simulink model "IntegratedControllerV9_WORKING"  (R2024b)
settings: Solver=FixedStepDiscrete  StartTime=0.0  StopTime=inf  FixedStep=0.01  RelTol=1e-3  EnableMultiTasking=on
model workspace (MAT data in the model file):
  kp = 1
undefined symbols (not defined in the file): a, b, dspDeleteFVToolLinkFromMask, gcbh
libraries: raspberrypiBasiclib x6, slpidlib x5, simulink x3, raspberrypiIOTlib x3, dspstat3 x2, etargetslib x2, eeGeneralControl x2, dspfiltersrcs x1
settings Model: ExtModeTrigDuration=2  Creator=alexs  LastModifiedBy=alexs
settings SolverCC: PositivePriorityOrder=on
settings OptimizationCC: EnhancedBackFolding=on  PassReuseOutputArgsAs=Individual arguments  ZeroExternalMemoryAtStartup=off  ZeroInternalMemoryAtStartup=off  MaxStackSize=200000  OptimizeBlockOrder=speed  DifferentSizesBufferReuse=on  EfficientTunableParamExpr=on
settings DebuggingCC: ParameterTunabilityLossMsg=error
settings HardwareCC: ProdBitPerPointer=32  ProdBitPerSizeT=32  ProdBitPerPtrDiffT=32  ProdLargestAtomicInteger=Long  ProdLargestAtomicFloat=Double  ProdWordSize=32  ProdLongLongMode=on  ProdHWDeviceType=ARM Compatible->ARM Cortex-A (32-bit)
settings RTWCC: Description=Embedded Coder  SystemTargetFile=ert.tlc  HardwareBoard=Raspberry Pi  TLCOptions="-aInlineSetEventsForThisBaseRateFcn=TLC_FALSE -aSuppressMultiTaskScheduler=TLC_FALSE  -aRateBasedStepFcn=0"  TemplateMakefile=ert_default_tmf  Toolchain=GNU GCC Embedded Linux  BuildConfiguration=Faster Runs
settings CodeAppCC: ForceParamTrailComments=on  IgnoreCustomStorageClasses=off  OperatorAnnotations=on  SimulinkDataObjDesc=on  SFDataObjDesc=on  InsertBlockDesc=on
settings ERTTargetCC: CodeReplacementLibrary=ARM Cortex-A CMSIS  SupportVariableSizeSignals=on  ExtModeTransport=2  ExtModeStaticAlloc=on  ExtModeMexFile=ext_xcp  ExtModeIntrfLevel=Level2 - Open  InlinedParameterPlacement=Hierarchical

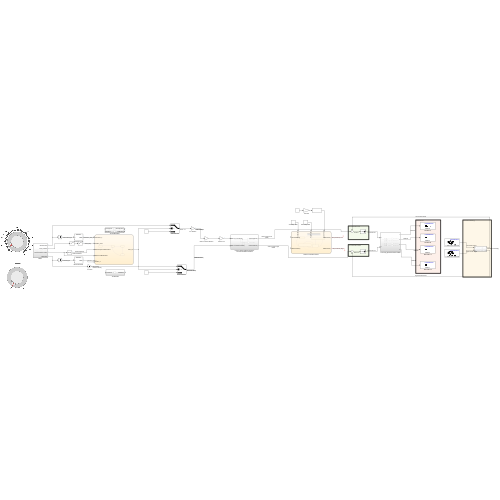
[thumbnail: Simulink's stored preview of the top-level diagram]
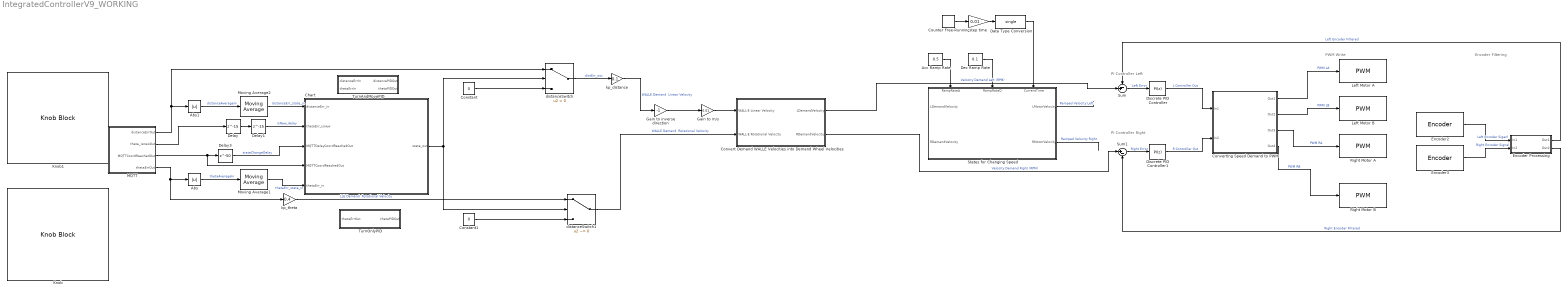
== system IntegratedControllerV9_WORKING ==
  note: PI Controller Right
  note: PWM Write
  note: PI Controller Left
  note: Encoder Filtering
  Abs : Abs  SaturateOnIntegerOverflow=off
  Abs1 : Abs  SaturateOnIntegerOverflow=off
  Acc Ramp Rate : Constant  Value=0.5  OutDataTypeStr=single
  Chart : Stateflow chart  TreatAsAtomicUnit=on
      settings: PortSchema="{\"entries\":[{\"content\":{\"sides\":[{\"content\":{\"connectorIds\":[\"In2\",\"In5\",\"In4\",\"In3\",\"In1\"]},\"type\":\"ConnectorPlacement.EquallySpacedRectSide\",\"uuid\":\"3dab0a91-9335-4990-9001-e160d82c945d\"},{\"content\":{\"connectorIds\":[\"Out1\"],\"side\":\"RIGHT\"},\"type\":\"ConnectorPlacement.EquallySpacedRectSide\",\"uuid\":\"b7b74537-0e0f-4d24-ad6a-0417436d6279\"},{\"content\":{\"side\":\"TOP\"},\"type\":\"ConnectorPlacement.EquallySpacedRectSide\",\"uuid\":\"7a696c29-7520-49e4-ace4-9e1abb82cb02\"}]},\"type\":\"ConnectorPlacement.EquallySpacedConnector\",\"uuid\":\"f02ffd70-1b39-4b11-b25b-86965795cc2a\"}],\"packageUris\":[\"http://schema.mathworks.com/mf0/Connector/R2020b\"],\"version\":\"1.0\"}"
  Constant : Constant  Value=0
  Constant1 : Constant  Value=0
  Convert Demand WALLE Velocities into Demand Wheel Velocities : Subsystem
  Converting Speed Demand to PWM : Subsystem
  Counter Free-Running : simulink/Sources/Counter Free-Running  NumBits=16  tsamp=-1
  Data Type Conversion : DataTypeConversion  OutDataTypeStr=single  SaturateOnIntegerOverflow=off  RndMeth=Floor
  Dec Ramp Rate : Constant  Value=0.1  OutDataTypeStr=single
  Delay : Delay  DelayLength=15  InitialCondition=0
  Delay1 : Delay  DelayLength=15  InitialCondition=0
  Delay3 : Delay  DelayLength=50  InitialCondition=0
  Discrete PID Controller : slpidlib/PID Controller  Controller=PI  Form=Parallel  TimeDomain=Discrete-time  UseExternalTs=off  SampleTime=-1  IntegratorMethod=Forward Euler  FilterMethod=Forward Euler  ControllerParametersSource=internal  P=1.7  I=0.4  UseKiTs=off  D=0.001  UseExternalDerivativeSource=off  N=100  UseFilter=on  TunerSelectOption=Transfer Function Based (PID Tuner App)  InitialConditionSource=internal  InitialConditionForIntegrator=0  InitialConditionForFilter=0  DifferentiatorICPrevScaledInput=0  ExternalReset=none  TrackingMode=off  Kt=1  LimitOutput=on  SatLimitsSource=internal  UpperSaturationLimit=44  LowerSaturationLimit=-44  LinearizeAsGain=off  AntiWindupMode=none  Kb=1  LimitIntegrator=off  UpperIntegratorSaturationLimit=inf  LowerIntegratorSaturationLimit=-inf  POutMin=[]  POutMax=[]  IOutMin=[]  IOutMax=[]  DOutMin=[]  DOutMax=[]  NOutMin=[]  NOutMax=[]  SumOutDataTypeStr=single  SumOutMin=[]  SumOutMax=[]  SaturationOutMin=[]  SaturationOutMax=[]  PParamMin=[]  PParamMax=[]  IParamMin=[]  IParamMax=[]  DParamMin=[]  DParamMax=[]  NParamMin=[]  NParamMax=[]  KbParamMin=[]  KbParamMax=[]  KtParamMin=[]  KtParamMax=[]  KbOutMin=[]  KbOutMax=[]  KtOutMin=[]  KtOutMax=[]  IntegratorOutMin=[]  IntegratorOutMax=[]  FilterOutMin=[]  FilterOutMax=[]  SumI1OutMin=[]  SumI1OutMax=[]  SumI2OutMin=[]  SumI2OutMax=[]  SumI3OutMin=[]  SumI3OutMax=[]  SumI4OutMin=[]  SumI4OutMax=[]  SumDOutMin=[]  SumDOutMax=[]  DifferentiatorOutMin=[]  DifferentiatorOutMax=[]  FilterDiffOutCoefMin=[]  FilterDiffOutCoefMax=[]  ReciprocalOutMin=[]  ReciprocalOutMax=[]  SumDenOutMin=[]  SumDenOutMax=[]  SumNumOutMin=[]  SumNumOutMax=[]  DivideOutMin=[]  DivideOutMax=[]  UdiffTsProdOutMin=[]  UdiffTsProdOutMax=[]  NTsProdOutMin=[]  NTsProdOutMax=[]  UintegralTsProdOutMin=[]  UintegralTsProdOutMax=[]  UngainTsProdOutMin=[]  UngainTsProdOutMax=[]  ClampingZeroOutDataTypeStr=Inherit: Inherit via back propagation  ClampingZeroOutMin=[]  ClampingZeroOutMax=[]  FilterDenConstantOutDataTypeStr=Inherit: Inherit via back propagation  FilterDenConstantOutMin=[]  FilterDenConstantOutMax=[]  PCopyOutDataTypeStr=Inherit: Inherit via back propagation  PCopyOutMin=[]  PCopyOutMax=[]  NCopyOutDataTypeStr=Inherit: Inherit via back propagation  NCopyOutMin=[]  NCopyOutMax=[]  IntegratorContinuousStateAttributes=''  IntegratorStateMustResolveToSignalObject=off  IntegratorRTWStateStorageClass=Auto  FilterContinuousStateAttributes=''  FilterStateMustResolveToSignalObject=off  FilterRTWStateStorageClass=Auto  ParallelPVariant=InternalParameters  IdealPVariant=Disabled  IVariant=InternalParameters  DVariant=Disabled  IntegratorVariant=Discrete  SatVariant=Enabled  AWVariant=Passthrough  PCopyVariant=Disabled  TRVariant=Disabled  FdbkBlocksVariant=Forward  IdealPFdbkVariant=Disabled  SatFdbkVariant=Disabled  DerivativeFilterVariant=Disabled  NVariant=Disabled  NCopyVariant=Disabled_SignalSpec  FilterICVariant=Disabled  IntegratorICVariant=InternalICs  ExternalResetVariant=Disabled  TRSumVariant=Passthrough  SumFdbkVariant=Disabled  SumVariant=Sum_PI  TsampFilterVariant=InternalTs  TsampNgainVariant=Passthrough  TsampIntegralVariant=Disabled_SignalSpec  ExternalSaturationOutDataTypeStr=Inherit: Same as second input  DerivativeSourceVariant=Disabled  PreIntVariant=InternalPreInt
      settings: LibrarySourceBlock=simulink/Discrete/Discrete PID Controller
  Discrete PID Controller1 : slpidlib/PID Controller  Controller=PI  Form=Parallel  TimeDomain=Discrete-time  UseExternalTs=off  SampleTime=-1  IntegratorMethod=Forward Euler  FilterMethod=Forward Euler  ControllerParametersSource=internal  P=1.7  I=0.4  UseKiTs=off  D=0  UseExternalDerivativeSource=off  N=100  UseFilter=on  TunerSelectOption=Transfer Function Based (PID Tuner App)  InitialConditionSource=internal  InitialConditionForIntegrator=0  InitialConditionForFilter=0  DifferentiatorICPrevScaledInput=0  ExternalReset=none  TrackingMode=off  Kt=1  LimitOutput=on  SatLimitsSource=internal  UpperSaturationLimit=44  LowerSaturationLimit=-44  LinearizeAsGain=off  AntiWindupMode=none  Kb=1  LimitIntegrator=off  UpperIntegratorSaturationLimit=inf  LowerIntegratorSaturationLimit=-inf  POutMin=[]  POutMax=[]  IOutMin=[]  IOutMax=[]  DOutMin=[]  DOutMax=[]  NOutMin=[]  NOutMax=[]  SumOutMin=[]  SumOutMax=[]  SaturationOutMin=[]  SaturationOutMax=[]  PParamMin=[]  PParamMax=[]  IParamMin=[]  IParamMax=[]  DParamMin=[]  DParamMax=[]  NParamMin=[]  NParamMax=[]  KbParamMin=[]  KbParamMax=[]  KtParamMin=[]  KtParamMax=[]  KbOutMin=[]  KbOutMax=[]  KtOutMin=[]  KtOutMax=[]  IntegratorOutMin=[]  IntegratorOutMax=[]  FilterOutMin=[]  FilterOutMax=[]  SumI1OutMin=[]  SumI1OutMax=[]  SumI2OutMin=[]  SumI2OutMax=[]  SumI3OutMin=[]  SumI3OutMax=[]  SumI4OutMin=[]  SumI4OutMax=[]  SumDOutMin=[]  SumDOutMax=[]  DifferentiatorOutMin=[]  DifferentiatorOutMax=[]  FilterDiffOutCoefMin=[]  FilterDiffOutCoefMax=[]  ReciprocalOutMin=[]  ReciprocalOutMax=[]  SumDenOutMin=[]  SumDenOutMax=[]  SumNumOutMin=[]  SumNumOutMax=[]  DivideOutMin=[]  DivideOutMax=[]  UdiffTsProdOutMin=[]  UdiffTsProdOutMax=[]  NTsProdOutMin=[]  NTsProdOutMax=[]  UintegralTsProdOutMin=[]  UintegralTsProdOutMax=[]  UngainTsProdOutMin=[]  UngainTsProdOutMax=[]  ClampingZeroOutDataTypeStr=Inherit: Inherit via back propagation  ClampingZeroOutMin=[]  ClampingZeroOutMax=[]  FilterDenConstantOutDataTypeStr=Inherit: Inherit via back propagation  FilterDenConstantOutMin=[]  FilterDenConstantOutMax=[]  PCopyOutDataTypeStr=Inherit: Inherit via back propagation  PCopyOutMin=[]  PCopyOutMax=[]  NCopyOutDataTypeStr=Inherit: Inherit via back propagation  NCopyOutMin=[]  NCopyOutMax=[]  IntegratorContinuousStateAttributes=''  IntegratorStateMustResolveToSignalObject=off  IntegratorRTWStateStorageClass=Auto  FilterContinuousStateAttributes=''  FilterStateMustResolveToSignalObject=off  FilterRTWStateStorageClass=Auto  ParallelPVariant=InternalParameters  IdealPVariant=Disabled  IVariant=InternalParameters  DVariant=Disabled  IntegratorVariant=Discrete  SatVariant=Enabled  AWVariant=Passthrough  PCopyVariant=Disabled  TRVariant=Disabled  FdbkBlocksVariant=Forward  IdealPFdbkVariant=Disabled  SatFdbkVariant=Disabled  DerivativeFilterVariant=Disabled  NVariant=Disabled  NCopyVariant=Disabled_SignalSpec  FilterICVariant=Disabled  IntegratorICVariant=InternalICs  ExternalResetVariant=Disabled  TRSumVariant=Passthrough  SumFdbkVariant=Disabled  SumVariant=Sum_PI  TsampFilterVariant=InternalTs  TsampNgainVariant=Passthrough  TsampIntegralVariant=Disabled_SignalSpec  ExternalSaturationOutDataTypeStr=Inherit: Same as second input  DerivativeSourceVariant=Disabled  PreIntVariant=InternalPreInt
      settings: LibrarySourceBlock=simulink/Discrete/Discrete PID Controller
  Encoder Processing : Subsystem
  Encoder2 : raspberrypiBasiclib/Encoder  BoardProperty=Pi 3 Model B+  InputA=GPIO 16  InputB=GPIO 20  Mode=No reset  SampleTime=-1
  Encoder3 : raspberrypiBasiclib/Encoder  BoardProperty=Pi 3 Model B+  InputA=GPIO 19  InputB=GPIO 26  Mode=No reset  SampleTime=-1
  Gain to inverse direction : Gain  Gain=-1
  Gain to m/s : Gain  Gain=0.01
  Knob : KnobBlock  ScaleMin=0.4  ScaleMax=0.8  ScaleType=Log
  Knob1 : KnobBlock  ScaleMax=1
  Left Motor A : raspberrypiBasiclib/PWM  board=Pi 3 Model B+  Pin_=18  Frequency=4000  blockPlatform=Raspberry Pi
  Left Motor B : raspberrypiBasiclib/PWM  board=Pi 3 Model B+  Pin_=14  Frequency=4000  blockPlatform=Raspberry Pi
  MQTT : Subsystem
  Moving Average1 : eeGeneralControl/Moving Average  VariantControl=Variant1  LabelModeActiveChoice=Discrete  f=1  x0=10  BufferSize=8192  Ts=-1
      settings: LibrarySourceBlock=ee_sl_lib/General Control/Moving Average
  Moving Average2 : eeGeneralControl/Moving Average  VariantControl=Variant1  LabelModeActiveChoice=Discrete  f=1  x0=10  BufferSize=8192  Ts=-1
      settings: LibrarySourceBlock=ee_sl_lib/General Control/Moving Average
  Right Motor A : raspberrypiBasiclib/PWM  board=Pi 3 Model B+  Pin_=27  Frequency=4000  blockPlatform=Raspberry Pi
  Right Motor B : raspberrypiBasiclib/PWM  board=Pi 3 Model B+  Pin_=17  Frequency=4000  blockPlatform=Raspberry Pi
  States for Changing Speed : Stateflow chart  TreatAsAtomicUnit=on
      settings: PortSchema="{\"entries\":[{\"content\":{\"sides\":[{\"content\":{\"connectorIds\":[\"In1\",\"In2\"]},\"type\":\"ConnectorPlacement.EquallySpacedRectSide\",\"uuid\":\"29566149-d476-48be-bb8d-fc9ab2ff4a55\"},{\"content\":{\"connectorIds\":[\"Out1\",\"Out2\"],\"side\":\"RIGHT\"},\"type\":\"ConnectorPlacement.EquallySpacedRectSide\",\"uuid\":\"f908ad7a-2ba5-4204-8f83-b7448630d8f9\"},{\"content\":{\"connectorIds\":[\"In3\",\"In4\",\"In5\"],\"side\":\"TOP\"},\"type\":\"ConnectorPlacement.EquallySpacedRectSide\",\"uuid\":\"1bf600d9-c304-4bcd-9fe1-9d209939bb1c\"}]},\"type\":\"ConnectorPlacement.EquallySpacedConnector\",\"uuid\":\"d153a689-9e68-4d3b-a6cb-2781800d561b\"}],\"packageUris\":[\"http://schema.mathworks.com/mf0/Connector/R2020b\"],\"version\":\"1.0\"}"
  Sum : Sum  Inputs=-+|
  Sum1 : Sum  Inputs=|+-
  TurnAndMovePID : Subsystem
  TurnOnlyPID : Subsystem
  distanceSwitch : Switch  Criteria=u2 > Threshold  SaturateOnIntegerOverflow=off  InputSameDT=off
  distanceSwitch1 : Switch  Criteria=u2 ~= 0  SaturateOnIntegerOverflow=off  InputSameDT=off
  kp_distance : Gain  Gain=0.1
  kp_theta : Gain  Gain=0.4
  step time : Gain  Gain=0.01
  wires:
  distanceSwitch1/1 -> Convert Demand WALLE Velocities into Demand Wheel Velocities/2(WALL-E Rotational Velocity)  "WALLE Demand  Rotational Velocity"
  Discrete PID Controller/1 -> Converting Speed Demand to PWM/1(In1)  "L Controller Out"
  Converting Speed Demand to PWM/1(Out1) -> Left Motor A/1  "PWM LA"
  Encoder3/1 -> Encoder Processing/2(In2)  "Right Encoder Signal"
  Counter Free-Running/1 -> step time/1
  Sum1/1 -> Discrete PID Controller1/1  "Right Error"
  step time/1 -> Data Type Conversion/1
  States for Changing Speed/2(RMotorVelocity) -> ?  "Ramped Velocity Right"
  Converting Speed Demand to PWM/3(Out3) -> Right Motor A/1  "PWM RA"
  Encoder2/1 -> Encoder Processing/1(In1)  "Left Encoder Siganl"
  Encoder Processing/2(Out2) -> Sum1/2  "Right Encoder Filtered"
  Discrete PID Controller1/1 -> Converting Speed Demand to PWM/2(In2)  "R Controller Out"
  kp_distance/1 -> Gain to inverse direction/1  "WALLE Demand  Linear Velocity"
  Sum/1 -> Discrete PID Controller/1  "Left Error"
  Converting Speed Demand to PWM/4(Out4) -> Right Motor B/1  "PWM RB"
  Acc Ramp Rate/1 -> States for Changing Speed/3(RampRateA)
  Data Type Conversion/1 -> States for Changing Speed/5(CurrentTime)
  States for Changing Speed/1(LMotorVelocity) -> ?  "Ramped Velocity Left"
  Convert Demand WALLE Velocities into Demand Wheel Velocities/1(LDemandVelocity) -> Sum/2  "Velocity Demand Left (RPM)"
  Encoder Processing/1(Out1) -> Sum/1  "Left Encoder Filtered"
  Converting Speed Demand to PWM/2(Out2) -> Left Motor B/1  "PWM LB"
  Dec Ramp Rate/1 -> States for Changing Speed/4(RampRateD)
  Convert Demand WALLE Velocities into Demand Wheel Velocities/2(RDemandVelocity) -> Sum1/1  "Velocity Demand Right (RPM)"
  MQTT/1(distanceErrOut) -> distanceSwitch/1, Abs1/1
  Constant/1 -> distanceSwitch/3
  MQTT/4(thetaErrOut) -> Abs/1, kp_theta/1
  Chart/1(state_out) -> distanceSwitch1/2, distanceSwitch/2
  Abs1/1 -> Moving Average2/1  "distanceAverageIn"
  Abs/1 -> Moving Average1/1  "thetaAverageIn"
  distanceSwitch/1 -> kp_distance/1  "distErr_out"
  Moving Average1/1 -> Chart/1(thetaErr_in)  "thetaErr_state_in"
  Moving Average2/1 -> Chart/2(distanceErr_in)  "distanceErr_state_in"
  Delay/1 -> Delay1/1
  MQTT/2(theta_isnewOut) -> Delay/1
  Delay1/1 -> Chart/5(thetaErr_isnew)  "isNew_delay"
  Gain to inverse direction/1 -> Gain to m/s/1
  Gain to m/s/1 -> Convert Demand WALLE Velocities into Demand Wheel Velocities/1(WALL-E Linear Velocity)
  kp_theta/1 -> distanceSwitch1/1  "LLE Demand  Rotational Velocity"
  Constant1/1 -> distanceSwitch1/3
  MQTT/3(MQTTCoordReachedOut) -> Chart/3(MQTTCoordReachedOut), Delay3/1
  Delay3/1 -> Chart/4(MQTTDelayCoordReachedOut)  "stateChangeDelay"

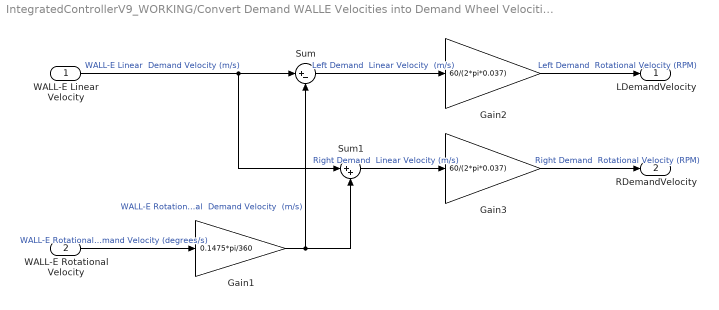
== system IntegratedControllerV9_WORKING/Convert Demand WALLE Velocities into Demand Wheel Velocities ==
  WALL-E Linear Velocity : Inport
  WALL-E Rotational Velocity : Inport  Port=2
  Gain1 : Gain  Gain=0.1475*pi/360
  Gain2 : Gain  Gain=60/(2*pi*0.037)
  Gain3 : Gain  Gain=60/(2*pi*0.037)
  Sum : Sum  Inputs=|+-  OutDataTypeStr=single
  Sum1 : Sum  Inputs=|++  OutDataTypeStr=single
  LDemandVelocity : Outport
  RDemandVelocity : Outport  Port=2
  wires:
  WALL-E Linear Velocity/1 -> Sum1/1, Sum/1  "WALL-E Linear  Demand Velocity (m/s)"
  WALL-E Rotational Velocity/1 -> Gain1/1  "WALL-E Rotational  Demand Velocity (degrees/s)"
  Gain1/1 -> Sum1/2, Sum/2  "WALL-E Rotational  Demand Velocity  (m/s)"
  Sum/1 -> Gain2/1  "Left Demand  Linear Velocity  (m/s)"
  Gain2/1 -> LDemandVelocity/1  "Left Demand  Rotational Velocity (RPM)"
  Sum1/1 -> Gain3/1  "Right Demand  Linear Velocity (m/s)"
  Gain3/1 -> RDemandVelocity/1  "Right Demand  Rotational Velocity (RPM)"

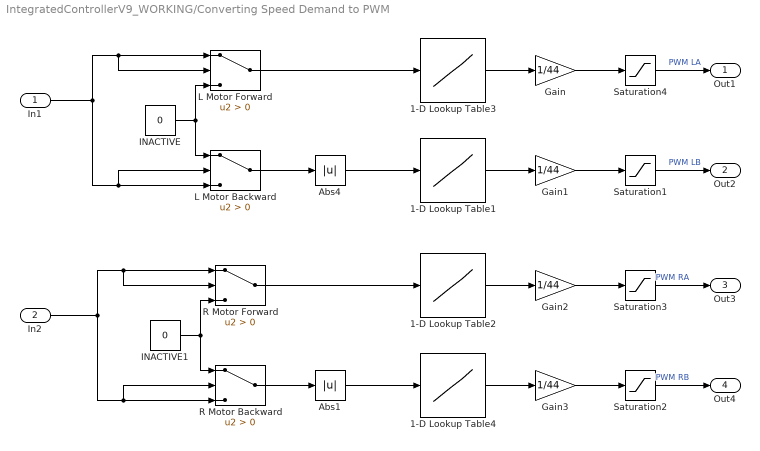
== system IntegratedControllerV9_WORKING/Converting Speed Demand to PWM ==
  In1 : Inport
  In2 : Inport  Port=2
  1-D Lookup Table{1..4} (4 alike) : Lookup_n-D  NumberOfTableDimensions=1  BreakpointsForDimension1=[0 2.1000000000000001 3.7000000000000002 5 10 15 20 25 30 35 40]  Table=[0 0 3.7000000000000002 3.7999999999999998 5 6 7 8 9 12 25]  InternalRulePriority=Speed  RndMeth=Simplest
  Abs1 : Abs  SaturateOnIntegerOverflow=off
  Abs4 : Abs  SaturateOnIntegerOverflow=off
  Gain{,1..3} (4 alike) : Gain  Gain=1/44
  INACTIVE : Constant  Value=0
  INACTIVE1 : Constant  Value=0
  L Motor Backward : Switch  Criteria=u2 > Threshold  SaturateOnIntegerOverflow=off  InputSameDT=off
  L Motor Forward : Switch  Criteria=u2 > Threshold  SaturateOnIntegerOverflow=off  InputSameDT=off
  R Motor Backward : Switch  Criteria=u2 > Threshold  SaturateOnIntegerOverflow=off  InputSameDT=off
  R Motor Forward : Switch  Criteria=u2 > Threshold  SaturateOnIntegerOverflow=off  InputSameDT=off
  Saturation{1..4} (4 alike) : Saturate  UpperLimit=1  LowerLimit=0
  Out1 : Outport
  Out2 : Outport  Port=2
  Out3 : Outport  Port=3
  Out4 : Outport  Port=4
  wires:
  L Motor Forward/1 -> 1-D Lookup Table3/1
  In1/1 -> L Motor Backward/2, L Motor Backward/3, L Motor Forward/2, L Motor Forward/1
  INACTIVE/1 -> L Motor Forward/3, L Motor Backward/1
  INACTIVE1/1 -> R Motor Forward/3, R Motor Backward/1
  R Motor Backward/1 -> Abs1/1
  In2/1 -> R Motor Backward/2, R Motor Backward/3, R Motor Forward/2, R Motor Forward/1
  R Motor Forward/1 -> 1-D Lookup Table2/1
  Saturation1/1 -> Out2/1  "PWM LB"
  Abs4/1 -> 1-D Lookup Table1/1
  L Motor Backward/1 -> Abs4/1
  Saturation4/1 -> Out1/1  "PWM LA"
  Saturation3/1 -> Out3/1  "PWM RA"
  Abs1/1 -> 1-D Lookup Table4/1
  Saturation2/1 -> Out4/1  "PWM RB"
  1-D Lookup Table2/1 -> Gain2/1
  1-D Lookup Table1/1 -> Gain1/1
  1-D Lookup Table3/1 -> Gain/1
  1-D Lookup Table4/1 -> Gain3/1
  Gain/1 -> Saturation4/1
  Gain1/1 -> Saturation1/1
  Gain2/1 -> Saturation3/1
  Gain3/1 -> Saturation2/1

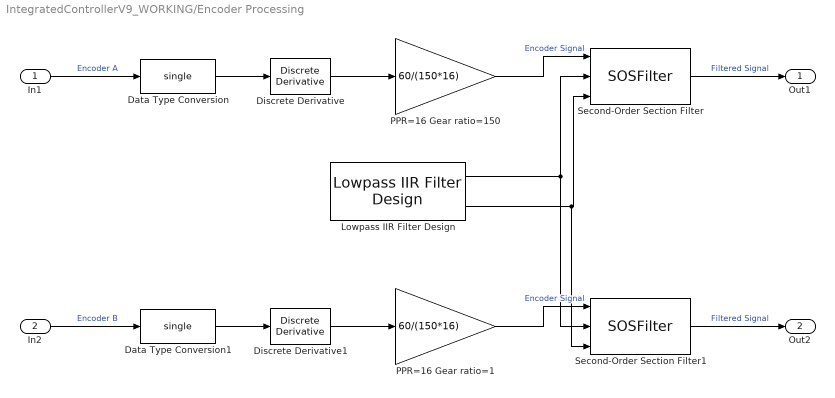
== system IntegratedControllerV9_WORKING/Encoder Processing ==
  In1 : Inport
  In2 : Inport  Port=2
  Data Type Conversion : DataTypeConversion  OutDataTypeStr=single  SaturateOnIntegerOverflow=off  RndMeth=Floor
  Data Type Conversion1 : DataTypeConversion  OutDataTypeStr=single  SaturateOnIntegerOverflow=off  RndMeth=Floor
  Discrete Derivative : simulink/Discrete/Discrete Derivative  gainval=1  ICPrevScaledInput=0.0  OutMin=[]  OutMax=[]  OutDataType=fixdt(1, 16)  OutScaling=2^-10  DoSatur=off
  Discrete Derivative1 : simulink/Discrete/Discrete Derivative  gainval=1  ICPrevScaledInput=0.0  OutMin=[]  OutMax=[]  OutDataType=fixdt(1, 16)  OutScaling=2^-10  DoSatur=off
  Lowpass IIR Filter Design : dspfiltersrcs/Lowpass IIR Filter Design  SmoothParameters=off  SmoothingFactor=0.6  DesignMethod=Butterworth  FilterOrderPort=off  FilterOrder=2  MaxOrder=2  F3dBPort=off  F3dB=50/200  ApassPort=off  Apass=1  AstopPort=off  Astop=60  HasScaleValues=off  OutputDataType=single  SampleTime=-1  SimulateUsing=Interpreted execution
  PPR=16 Gear ratio=1 : Gain  Gain=60/(150*16)  OutDataTypeStr=single
  PPR=16 Gear ratio=150 : Gain  Gain=60/(150*16)  OutDataTypeStr=single
  Second-Order Section Filter : SOSFilter  LoadFcn=dspDeleteFVToolLinkFromMask(gcbh);  CoeffSource=Input ports  Numerator=b  Denominator=a
      settings: DeleteFcn=dspLinkFVTool2Mask(gcbh,'close')  ModelCloseFcn=dspLinkFVTool2Mask(gcbh,'close')  PreSaveFcn=dspUnlinkFVToolFromMask(gcbh);  PostSaveFcn=dspRestoreLinkFVTool2Mask(gcbh);  CloseFcn=dspLinkFVTool2Mask(gcbh,'close')  InputPortMap=u0,u1,u2
      settings: CopyFcn=|
      | ud = get_param(gcbh,'UserData');
      | if isfield(ud,'fvtool')
      |   ud = rmfield(ud,'fvtool');
      |   set_param(gcbh,'UserData',ud);
      | end
      | clear ud
  Second-Order Section Filter1 : SOSFilter  LoadFcn=dspDeleteFVToolLinkFromMask(gcbh);  CoeffSource=Input ports  Numerator=b  Denominator=a
      settings: DeleteFcn=dspLinkFVTool2Mask(gcbh,'close')  ModelCloseFcn=dspLinkFVTool2Mask(gcbh,'close')  PreSaveFcn=dspUnlinkFVToolFromMask(gcbh);  PostSaveFcn=dspRestoreLinkFVTool2Mask(gcbh);  CloseFcn=dspLinkFVTool2Mask(gcbh,'close')  InputPortMap=u0,u1,u2
      settings: CopyFcn=|
      | ud = get_param(gcbh,'UserData');
      | if isfield(ud,'fvtool')
      |   ud = rmfield(ud,'fvtool');
      |   set_param(gcbh,'UserData',ud);
      | end
      | clear ud
  Out1 : Outport
  Out2 : Outport  Port=2
  wires:
  In1/1 -> Data Type Conversion/1  "Encoder A"
  Second-Order Section Filter/1 -> Out1/1  "Filtered Signal"
  Discrete Derivative/1 -> PPR=16 Gear ratio=150/1
  PPR=16 Gear ratio=150/1 -> Second-Order Section Filter/1  "Encoder Signal"
  Data Type Conversion/1 -> Discrete Derivative/1
  Lowpass IIR Filter Design/2 -> Second-Order Section Filter1/3, Second-Order Section Filter/3
  Data Type Conversion1/1 -> Discrete Derivative1/1
  PPR=16 Gear ratio=1/1 -> Second-Order Section Filter1/1  "Encoder Signal"
  Second-Order Section Filter1/1 -> Out2/1  "Filtered Signal"
  Discrete Derivative1/1 -> PPR=16 Gear ratio=1/1
  In2/1 -> Data Type Conversion1/1  "Encoder B"
  Lowpass IIR Filter Design/1 -> Second-Order Section Filter/2, Second-Order Section Filter1/2

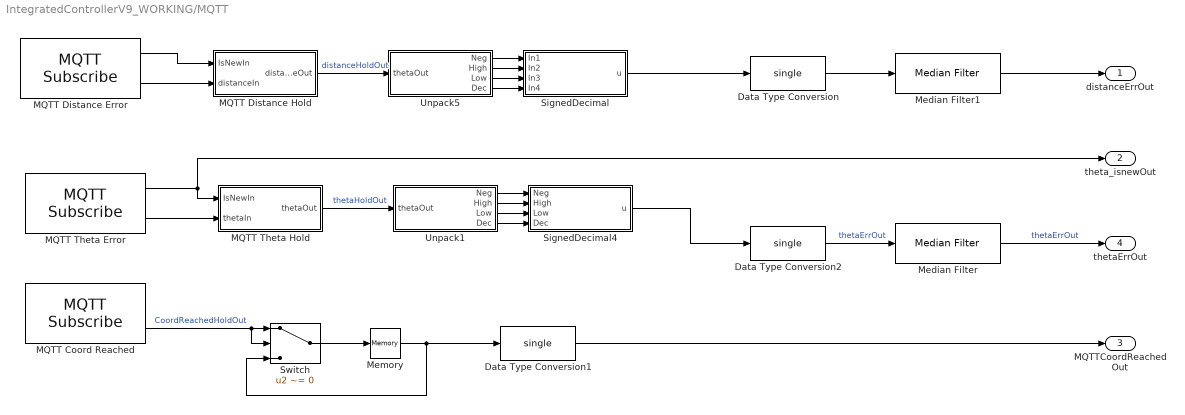
== system IntegratedControllerV9_WORKING/MQTT ==
  Data Type Conversion : DataTypeConversion  OutDataTypeStr=single  SaturateOnIntegerOverflow=off  RndMeth=Floor
  Data Type Conversion1 : DataTypeConversion  OutDataTypeStr=single  SaturateOnIntegerOverflow=off  RndMeth=Floor
  Data Type Conversion2 : DataTypeConversion  OutDataTypeStr=single  SaturateOnIntegerOverflow=off  RndMeth=Floor
  MQTT Coord Reached : raspberrypiIOTlib/MQTT Subscribe  Topic=Wall-E/position_controller/coord_reached  QoS=2  MessageLength=1  OutputMessage=on  SampleTime=.05  blockPlatform=RASPBERRYPI
  MQTT Distance Error : raspberrypiIOTlib/MQTT Subscribe  Topic=Wall-E/position_controller/error/dist  QoS=2  MessageLength=4  OutputMessage=on  SampleTime=.05  blockPlatform=RASPBERRYPI
  MQTT Distance Hold : Subsystem
  MQTT Theta Error : raspberrypiIOTlib/MQTT Subscribe  Topic=Wall-E/position_controller/error/theta  QoS=2  MessageLength=4  OutputMessage=on  SampleTime=.05  blockPlatform=RASPBERRYPI
  MQTT Theta Hold : Subsystem
  Median Filter : dspstat3/Median Filter  WindowLength=8  SimulateUsing=Interpreted execution
      settings: LibrarySourceBlock=|
      | dspfdesign/Median
      | Filter
  Median Filter1 : dspstat3/Median Filter  WindowLength=8  SimulateUsing=Interpreted execution
      settings: LibrarySourceBlock=|
      | dspfdesign/Median
      | Filter
  Memory : Memory  InheritSampleTime=on
  SignedDecimal : Subsystem
  SignedDecimal4 : Subsystem
  Switch : Switch  Criteria=u2 ~= 0  SaturateOnIntegerOverflow=off  InputSameDT=off
  Unpack1 : Subsystem
  Unpack5 : Subsystem
  distanceErrOut : Outport
  theta_isnewOut : Outport  Port=2
  MQTTCoordReachedOut : Outport  Port=3
  thetaErrOut : Outport  Port=4
  wires:
  Unpack5/4(Dec) -> SignedDecimal/4(In4)
  Unpack5/1(Neg) -> SignedDecimal/1(In1)
  Unpack5/2(High) -> SignedDecimal/2(In2)
  SignedDecimal/1(u) -> Data Type Conversion/1
  Unpack5/3(Low) -> SignedDecimal/3(In3)
  Median Filter1/1 -> distanceErrOut/1
  Unpack1/1(Neg) -> SignedDecimal4/1(Neg)
  Unpack1/2(High) -> SignedDecimal4/2(High)
  Unpack1/3(Low) -> SignedDecimal4/3(Low)
  Unpack1/4(Dec) -> SignedDecimal4/4(Dec)
  SignedDecimal4/1(u) -> Data Type Conversion2/1
  Median Filter/1 -> thetaErrOut/1  "thetaErrOut"
  MQTT Theta Error/1 -> theta_isnewOut/1, MQTT Theta Hold/1(IsNewIn)
  MQTT Theta Hold/1(thetaOut) -> Unpack1/1(thetaOut)  "thetaHoldOut"
  MQTT Theta Error/2 -> MQTT Theta Hold/2(thetaIn)
  MQTT Distance Hold/1(distanceOut) -> Unpack5/1(thetaOut)  "distanceHoldOut"
  MQTT Distance Error/2 -> MQTT Distance Hold/2(distanceIn)
  MQTT Distance Error/1 -> MQTT Distance Hold/1(IsNewIn)
  Data Type Conversion2/1 -> Median Filter/1  "thetaErrOut"
  Data Type Conversion/1 -> Median Filter1/1
  Switch/1 -> Memory/1
  Memory/1 -> Data Type Conversion1/1, Switch/3
  MQTT Coord Reached/2 -> Switch/2, Switch/1  "CoordReachedHoldOut"
  Data Type Conversion1/1 -> MQTTCoordReachedOut/1

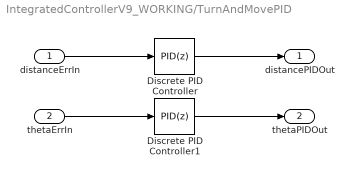
== system IntegratedControllerV9_WORKING/TurnAndMovePID ==
  distanceErrIn : Inport
  thetaErrIn : Inport  Port=2
  Discrete PID Controller : slpidlib/PID Controller  Controller=PID  Form=Parallel  TimeDomain=Discrete-time  UseExternalTs=off  SampleTime=0.25  IntegratorMethod=Forward Euler  FilterMethod=Forward Euler  ControllerParametersSource=internal  P=0.01  I=0  UseKiTs=off  D=.001  UseExternalDerivativeSource=off  N=100  UseFilter=on  TunerSelectOption=Transfer Function Based (PID Tuner App)  InitialConditionSource=internal  InitialConditionForIntegrator=0  InitialConditionForFilter=0  DifferentiatorICPrevScaledInput=0  ExternalReset=none  TrackingMode=off  Kt=1  LimitOutput=on  SatLimitsSource=internal  UpperSaturationLimit=1  LowerSaturationLimit=-1  LinearizeAsGain=off  AntiWindupMode=none  Kb=1  LimitIntegrator=off  UpperIntegratorSaturationLimit=inf  LowerIntegratorSaturationLimit=-inf  POutMin=[]  POutMax=[]  IOutMin=[]  IOutMax=[]  DOutMin=[]  DOutMax=[]  NOutMin=[]  NOutMax=[]  SumOutMin=[]  SumOutMax=[]  SaturationOutMin=[]  SaturationOutMax=[]  PParamMin=[]  PParamMax=[]  IParamMin=[]  IParamMax=[]  DParamMin=[]  DParamMax=[]  NParamMin=[]  NParamMax=[]  KbParamMin=[]  KbParamMax=[]  KtParamMin=[]  KtParamMax=[]  KbOutMin=[]  KbOutMax=[]  KtOutMin=[]  KtOutMax=[]  IntegratorOutMin=[]  IntegratorOutMax=[]  FilterOutMin=[]  FilterOutMax=[]  SumI1OutMin=[]  SumI1OutMax=[]  SumI2OutMin=[]  SumI2OutMax=[]  SumI3OutMin=[]  SumI3OutMax=[]  SumI4OutMin=[]  SumI4OutMax=[]  SumDOutMin=[]  SumDOutMax=[]  DifferentiatorOutMin=[]  DifferentiatorOutMax=[]  FilterDiffOutCoefMin=[]  FilterDiffOutCoefMax=[]  ReciprocalOutMin=[]  ReciprocalOutMax=[]  SumDenOutMin=[]  SumDenOutMax=[]  SumNumOutMin=[]  SumNumOutMax=[]  DivideOutMin=[]  DivideOutMax=[]  UdiffTsProdOutMin=[]  UdiffTsProdOutMax=[]  NTsProdOutMin=[]  NTsProdOutMax=[]  UintegralTsProdOutMin=[]  UintegralTsProdOutMax=[]  UngainTsProdOutMin=[]  UngainTsProdOutMax=[]  ClampingZeroOutDataTypeStr=Inherit: Inherit via back propagation  ClampingZeroOutMin=[]  ClampingZeroOutMax=[]  FilterDenConstantOutDataTypeStr=Inherit: Inherit via back propagation  FilterDenConstantOutMin=[]  FilterDenConstantOutMax=[]  PCopyOutDataTypeStr=Inherit: Inherit via back propagation  PCopyOutMin=[]  PCopyOutMax=[]  NCopyOutDataTypeStr=Inherit: Inherit via back propagation  NCopyOutMin=[]  NCopyOutMax=[]  IntegratorContinuousStateAttributes=''  IntegratorStateMustResolveToSignalObject=off  IntegratorRTWStateStorageClass=Auto  FilterContinuousStateAttributes=''  FilterStateMustResolveToSignalObject=off  FilterRTWStateStorageClass=Auto  ParallelPVariant=InternalParameters  IdealPVariant=Disabled  IVariant=InternalParameters  DVariant=InternalParameters  IntegratorVariant=Discrete  SatVariant=Enabled  AWVariant=Passthrough  PCopyVariant=Disabled  TRVariant=Disabled  FdbkBlocksVariant=Forward  IdealPFdbkVariant=Disabled  SatFdbkVariant=Disabled  DerivativeFilterVariant=ForwardEulerFilter  NVariant=InternalParameters  NCopyVariant=Disabled  FilterICVariant=InternalICsFilter  IntegratorICVariant=InternalICs  ExternalResetVariant=Disabled  TRSumVariant=Passthrough  SumFdbkVariant=Disabled  SumVariant=Sum_PID  TsampFilterVariant=InternalTs  TsampNgainVariant=Passthrough  TsampIntegralVariant=Disabled_SignalSpec  ExternalSaturationOutDataTypeStr=Inherit: Same as second input  DerivativeSourceVariant=ErrorSignal  PreIntVariant=InternalPreInt
  Discrete PID Controller1 : slpidlib/PID Controller  Controller=PID  Form=Parallel  TimeDomain=Discrete-time  UseExternalTs=off  SampleTime=0.25  IntegratorMethod=Forward Euler  FilterMethod=Forward Euler  ControllerParametersSource=internal  P=kp  I=1  UseKiTs=off  D=0  UseExternalDerivativeSource=off  N=100  UseFilter=on  TunerSelectOption=Transfer Function Based (PID Tuner App)  InitialConditionSource=internal  InitialConditionForIntegrator=0  InitialConditionForFilter=0  DifferentiatorICPrevScaledInput=0  ExternalReset=none  TrackingMode=off  Kt=1  LimitOutput=on  SatLimitsSource=internal  UpperSaturationLimit=90  LowerSaturationLimit=-90  LinearizeAsGain=off  AntiWindupMode=none  Kb=1  LimitIntegrator=off  UpperIntegratorSaturationLimit=inf  LowerIntegratorSaturationLimit=-inf  POutMin=[]  POutMax=[]  IOutMin=[]  IOutMax=[]  DOutMin=[]  DOutMax=[]  NOutMin=[]  NOutMax=[]  SumOutMin=[]  SumOutMax=[]  SaturationOutMin=[]  SaturationOutMax=[]  PParamMin=[]  PParamMax=[]  IParamMin=[]  IParamMax=[]  DParamMin=[]  DParamMax=[]  NParamMin=[]  NParamMax=[]  KbParamMin=[]  KbParamMax=[]  KtParamMin=[]  KtParamMax=[]  KbOutMin=[]  KbOutMax=[]  KtOutMin=[]  KtOutMax=[]  IntegratorOutMin=[]  IntegratorOutMax=[]  FilterOutMin=[]  FilterOutMax=[]  SumI1OutMin=[]  SumI1OutMax=[]  SumI2OutMin=[]  SumI2OutMax=[]  SumI3OutMin=[]  SumI3OutMax=[]  SumI4OutMin=[]  SumI4OutMax=[]  SumDOutMin=[]  SumDOutMax=[]  DifferentiatorOutMin=[]  DifferentiatorOutMax=[]  FilterDiffOutCoefMin=[]  FilterDiffOutCoefMax=[]  ReciprocalOutMin=[]  ReciprocalOutMax=[]  SumDenOutMin=[]  SumDenOutMax=[]  SumNumOutMin=[]  SumNumOutMax=[]  DivideOutMin=[]  DivideOutMax=[]  UdiffTsProdOutMin=[]  UdiffTsProdOutMax=[]  NTsProdOutMin=[]  NTsProdOutMax=[]  UintegralTsProdOutMin=[]  UintegralTsProdOutMax=[]  UngainTsProdOutMin=[]  UngainTsProdOutMax=[]  ClampingZeroOutDataTypeStr=Inherit: Inherit via back propagation  ClampingZeroOutMin=[]  ClampingZeroOutMax=[]  FilterDenConstantOutDataTypeStr=Inherit: Inherit via back propagation  FilterDenConstantOutMin=[]  FilterDenConstantOutMax=[]  PCopyOutDataTypeStr=Inherit: Inherit via back propagation  PCopyOutMin=[]  PCopyOutMax=[]  NCopyOutDataTypeStr=Inherit: Inherit via back propagation  NCopyOutMin=[]  NCopyOutMax=[]  IntegratorContinuousStateAttributes=''  IntegratorStateMustResolveToSignalObject=off  IntegratorRTWStateStorageClass=Auto  FilterContinuousStateAttributes=''  FilterStateMustResolveToSignalObject=off  FilterRTWStateStorageClass=Auto  ParallelPVariant=InternalParameters  IdealPVariant=Disabled  IVariant=InternalParameters  DVariant=InternalParameters  IntegratorVariant=Discrete  SatVariant=Enabled  AWVariant=Passthrough  PCopyVariant=Disabled  TRVariant=Disabled  FdbkBlocksVariant=Forward  IdealPFdbkVariant=Disabled  SatFdbkVariant=Disabled  DerivativeFilterVariant=ForwardEulerFilter  NVariant=InternalParameters  NCopyVariant=Disabled  FilterICVariant=InternalICsFilter  IntegratorICVariant=InternalICs  ExternalResetVariant=Disabled  TRSumVariant=Passthrough  SumFdbkVariant=Disabled  SumVariant=Sum_PID  TsampFilterVariant=InternalTs  TsampNgainVariant=Passthrough  TsampIntegralVariant=Disabled_SignalSpec  ExternalSaturationOutDataTypeStr=Inherit: Same as second input  DerivativeSourceVariant=ErrorSignal  PreIntVariant=InternalPreInt
  distancePIDOut : Outport
  thetaPIDOut : Outport  Port=2
  wires:
  distanceErrIn/1 -> Discrete PID Controller/1
  Discrete PID Controller/1 -> distancePIDOut/1
  Discrete PID Controller1/1 -> thetaPIDOut/1
  thetaErrIn/1 -> Discrete PID Controller1/1

== system IntegratedControllerV9_WORKING/TurnOnlyPID ==
  thetaErrOut : Inport
  Discrete PID Controller : slpidlib/PID Controller  Controller=PID  Form=Parallel  TimeDomain=Discrete-time  UseExternalTs=off  SampleTime=0.25  IntegratorMethod=Forward Euler  FilterMethod=Forward Euler  ControllerParametersSource=internal  P=kp  I=1  UseKiTs=off  D=.00001  UseExternalDerivativeSource=off  N=100  UseFilter=on  TunerSelectOption=Transfer Function Based (PID Tuner App)  InitialConditionSource=internal  InitialConditionForIntegrator=0  InitialConditionForFilter=0  DifferentiatorICPrevScaledInput=0  ExternalReset=none  TrackingMode=off  Kt=1  LimitOutput=on  SatLimitsSource=internal  UpperSaturationLimit=90  LowerSaturationLimit=-90  LinearizeAsGain=off  AntiWindupMode=none  Kb=1  LimitIntegrator=off  UpperIntegratorSaturationLimit=inf  LowerIntegratorSaturationLimit=-inf  POutMin=[]  POutMax=[]  IOutMin=[]  IOutMax=[]  DOutMin=[]  DOutMax=[]  NOutMin=[]  NOutMax=[]  SumOutMin=[]  SumOutMax=[]  SaturationOutMin=[]  SaturationOutMax=[]  PParamMin=[]  PParamMax=[]  IParamMin=[]  IParamMax=[]  DParamMin=[]  DParamMax=[]  NParamMin=[]  NParamMax=[]  KbParamMin=[]  KbParamMax=[]  KtParamMin=[]  KtParamMax=[]  KbOutMin=[]  KbOutMax=[]  KtOutMin=[]  KtOutMax=[]  IntegratorOutMin=[]  IntegratorOutMax=[]  FilterOutMin=[]  FilterOutMax=[]  SumI1OutMin=[]  SumI1OutMax=[]  SumI2OutMin=[]  SumI2OutMax=[]  SumI3OutMin=[]  SumI3OutMax=[]  SumI4OutMin=[]  SumI4OutMax=[]  SumDOutMin=[]  SumDOutMax=[]  DifferentiatorOutMin=[]  DifferentiatorOutMax=[]  FilterDiffOutCoefMin=[]  FilterDiffOutCoefMax=[]  ReciprocalOutMin=[]  ReciprocalOutMax=[]  SumDenOutMin=[]  SumDenOutMax=[]  SumNumOutMin=[]  SumNumOutMax=[]  DivideOutMin=[]  DivideOutMax=[]  UdiffTsProdOutMin=[]  UdiffTsProdOutMax=[]  NTsProdOutMin=[]  NTsProdOutMax=[]  UintegralTsProdOutMin=[]  UintegralTsProdOutMax=[]  UngainTsProdOutMin=[]  UngainTsProdOutMax=[]  ClampingZeroOutDataTypeStr=Inherit: Inherit via back propagation  ClampingZeroOutMin=[]  ClampingZeroOutMax=[]  FilterDenConstantOutDataTypeStr=Inherit: Inherit via back propagation  FilterDenConstantOutMin=[]  FilterDenConstantOutMax=[]  PCopyOutDataTypeStr=Inherit: Inherit via back propagation  PCopyOutMin=[]  PCopyOutMax=[]  NCopyOutDataTypeStr=Inherit: Inherit via back propagation  NCopyOutMin=[]  NCopyOutMax=[]  IntegratorContinuousStateAttributes=''  IntegratorStateMustResolveToSignalObject=off  IntegratorRTWStateStorageClass=Auto  FilterContinuousStateAttributes=''  FilterStateMustResolveToSignalObject=off  FilterRTWStateStorageClass=Auto  ParallelPVariant=InternalParameters  IdealPVariant=Disabled  IVariant=InternalParameters  DVariant=InternalParameters  IntegratorVariant=Discrete  SatVariant=Enabled  AWVariant=Passthrough  PCopyVariant=Disabled  TRVariant=Disabled  FdbkBlocksVariant=Forward  IdealPFdbkVariant=Disabled  SatFdbkVariant=Disabled  DerivativeFilterVariant=ForwardEulerFilter  NVariant=InternalParameters  NCopyVariant=Disabled  FilterICVariant=InternalICsFilter  IntegratorICVariant=InternalICs  ExternalResetVariant=Disabled  TRSumVariant=Passthrough  SumFdbkVariant=Disabled  SumVariant=Sum_PID  TsampFilterVariant=InternalTs  TsampNgainVariant=Passthrough  TsampIntegralVariant=Disabled_SignalSpec  ExternalSaturationOutDataTypeStr=Inherit: Same as second input  DerivativeSourceVariant=ErrorSignal  PreIntVariant=InternalPreInt
      settings: LibrarySourceBlock=simulink/Discrete/Discrete PID Controller
  thetaPIDOut : Outport
  wires:
  thetaErrOut/1 -> Discrete PID Controller/1
  Discrete PID Controller/1 -> thetaPIDOut/1

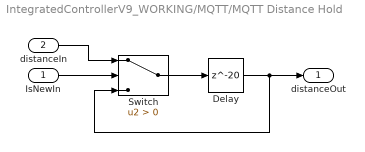
== system IntegratedControllerV9_WORKING/MQTT/MQTT Distance Hold ==
  IsNewIn : Inport
  distanceIn : Inport  Port=2
  Delay : Delay  DelayLength=20  InitialCondition=0
  Switch : Switch  Criteria=u2 > Threshold  SaturateOnIntegerOverflow=off  InputSameDT=off
  distanceOut : Outport
  wires:
  Delay/1 -> distanceOut/1, Switch/3
  Switch/1 -> Delay/1
  distanceIn/1 -> Switch/1
  IsNewIn/1 -> Switch/2

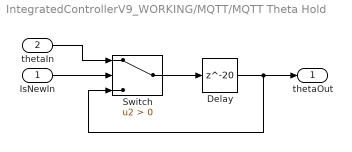
== system IntegratedControllerV9_WORKING/MQTT/MQTT Theta Hold ==
  IsNewIn : Inport
  thetaIn : Inport  Port=2
  Delay : Delay  DelayLength=20  InitialCondition=0
  Switch : Switch  Criteria=u2 > Threshold  SaturateOnIntegerOverflow=off  InputSameDT=off
  thetaOut : Outport
  wires:
  Delay/1 -> thetaOut/1, Switch/3
  Switch/1 -> Delay/1
  thetaIn/1 -> Switch/1
  IsNewIn/1 -> Switch/2

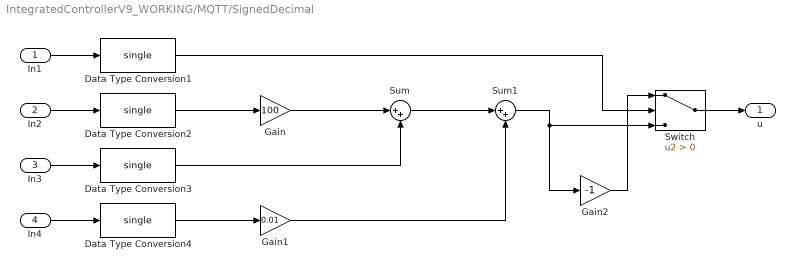
== system IntegratedControllerV9_WORKING/MQTT/SignedDecimal ==
  In1 : Inport
  In2 : Inport  Port=2
  In3 : Inport  Port=3
  In4 : Inport  Port=4
  Data Type Conversion{1..4} (4 alike) : DataTypeConversion  OutDataTypeStr=single  SaturateOnIntegerOverflow=off  RndMeth=Floor
  Gain : Gain  Gain=100
  Gain1 : Gain  Gain=0.01
  Gain2 : Gain  Gain=-1
  Sum : Sum  Inputs=|++
  Sum1 : Sum  Inputs=|++
  Switch : Switch  Criteria=u2 > Threshold  SaturateOnIntegerOverflow=off  InputSameDT=off
  u : Outport
  wires:
  Data Type Conversion4/1 -> Gain1/1
  Sum1/1 -> Switch/3, Gain2/1
  Sum/1 -> Sum1/1
  Gain1/1 -> Sum1/2
  Data Type Conversion1/1 -> Switch/2
  Gain/1 -> Sum/1
  Data Type Conversion3/1 -> Sum/2
  Switch/1 -> u/1
  Data Type Conversion2/1 -> Gain/1
  In1/1 -> Data Type Conversion1/1
  In2/1 -> Data Type Conversion2/1
  In3/1 -> Data Type Conversion3/1
  In4/1 -> Data Type Conversion4/1
  Gain2/1 -> Switch/1

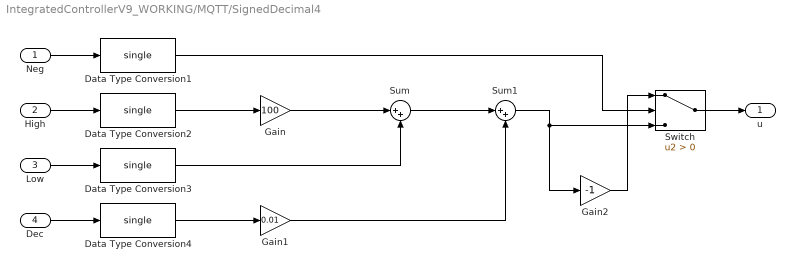
== system IntegratedControllerV9_WORKING/MQTT/SignedDecimal4 ==
  Neg : Inport
  High : Inport  Port=2
  Low : Inport  Port=3
  Dec : Inport  Port=4
  Data Type Conversion{1..4} (4 alike) : DataTypeConversion  OutDataTypeStr=single  SaturateOnIntegerOverflow=off  RndMeth=Floor
  Gain : Gain  Gain=100
  Gain1 : Gain  Gain=0.01
  Gain2 : Gain  Gain=-1
  Sum : Sum  Inputs=|++
  Sum1 : Sum  Inputs=|++
  Switch : Switch  Criteria=u2 > Threshold  SaturateOnIntegerOverflow=off  InputSameDT=off
  u : Outport
  wires:
  Data Type Conversion4/1 -> Gain1/1
  Sum1/1 -> Switch/3, Gain2/1
  Sum/1 -> Sum1/1
  Gain1/1 -> Sum1/2
  Data Type Conversion1/1 -> Switch/2
  Gain/1 -> Sum/1
  Data Type Conversion3/1 -> Sum/2
  Switch/1 -> u/1
  Data Type Conversion2/1 -> Gain/1
  Neg/1 -> Data Type Conversion1/1
  High/1 -> Data Type Conversion2/1
  Low/1 -> Data Type Conversion3/1
  Dec/1 -> Data Type Conversion4/1
  Gain2/1 -> Switch/1

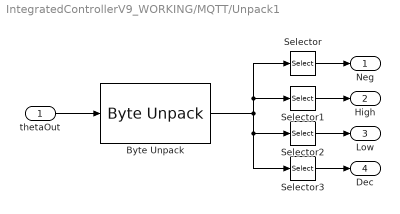
== system IntegratedControllerV9_WORKING/MQTT/Unpack1 ==
  thetaOut : Inport
  Byte Unpack : etargetslib/Byte Unpack  dimensions={[4]}  datatypes={'uint8'}  byteAlign=1
  Selector : Selector  InputPortWidth=4  IndexOptions=Index vector (dialog)  Indices=[1]  OutputSizes=1
  Selector1 : Selector  InputPortWidth=4  IndexOptions=Index vector (dialog)  Indices=[2]  OutputSizes=1
  Selector2 : Selector  InputPortWidth=4  IndexOptions=Index vector (dialog)  Indices=[3]  OutputSizes=1
  Selector3 : Selector  InputPortWidth=4  IndexOptions=Index vector (dialog)  Indices=[4]  OutputSizes=1
  Neg : Outport
  High : Outport  Port=2
  Low : Outport  Port=3
  Dec : Outport  Port=4
  wires:
  Byte Unpack/1 -> Selector1/1, Selector/1, Selector3/1, Selector2/1
  Selector/1 -> Neg/1
  Selector1/1 -> High/1
  Selector2/1 -> Low/1
  Selector3/1 -> Dec/1
  thetaOut/1 -> Byte Unpack/1

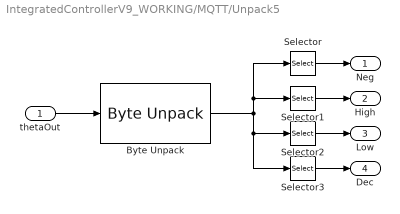
== system IntegratedControllerV9_WORKING/MQTT/Unpack5 ==
  thetaOut : Inport
  Byte Unpack : etargetslib/Byte Unpack  dimensions={[4]}  datatypes={'uint8'}  byteAlign=1
  Selector : Selector  InputPortWidth=4  IndexOptions=Index vector (dialog)  Indices=[1]  OutputSizes=1
  Selector1 : Selector  InputPortWidth=4  IndexOptions=Index vector (dialog)  Indices=[2]  OutputSizes=1
  Selector2 : Selector  InputPortWidth=4  IndexOptions=Index vector (dialog)  Indices=[3]  OutputSizes=1
  Selector3 : Selector  InputPortWidth=4  IndexOptions=Index vector (dialog)  Indices=[4]  OutputSizes=1
  Neg : Outport
  High : Outport  Port=2
  Low : Outport  Port=3
  Dec : Outport  Port=4
  wires:
  Byte Unpack/1 -> Selector1/1, Selector/1, Selector3/1, Selector2/1
  Selector/1 -> Neg/1
  Selector1/1 -> High/1
  Selector2/1 -> Low/1
  Selector3/1 -> Dec/1
  thetaOut/1 -> Byte Unpack/1

== stateflow chart IntegratedControllerV9_WORKING/Chart ==
  state TurnOnly
    en: state_out = -1
  state TurnAndMove
    en: state_out = 1
  state Idle
    en: state_out = 0
  note: Turning and going forwards
  note: Turning only here
  state AtTarget
    en: state_out = -2
  note: Turning only here
  (default) -> Idle
  Idle -> TurnOnly : [thetaErr_isnew ~= 0]
  TurnOnly -> TurnAndMove : [thetaErr_in < 10]
  AtTarget -> TurnOnly : [MQTTDelayCoordReachedOut == 2]
  TurnAndMove -> AtTarget : [MQTTCoordReachedOut == 1]
  data: thetaErr_in input; distanceErr_in input; MQTTCoordReachedOut input; MQTTDelayCoordReachedOut input; thetaErr_isnew input; state_out output

== stateflow chart IntegratedControllerV9_WORKING/States for Changing Speed ==
  state Idle
    en:
    LMotorVelocity = 0;
    RMotorVelocity = 0;
    StepTime = single(0);
  state Accelerating
    du:
    LMotorVelocity = stepToRamp(CurrentTime, StepTime, LDemandVelocity, LMotorVelocity, RampRateA);
    RMotorVelocity = stepToRamp(CurrentTime, StepTime, RDemandVelocity, RMotorVelocity, RampRateA);
  state Decelerating
    du:
    LMotorVelocity = stepToRamp(CurrentTime, StepTime, LDemandVelocity, LMotorVelocity, RampRateD);
    RMotorVelocity = stepToRamp(CurrentTime, StepTime, RDemandVelocity, RMotorVelocity, RampRateD);
  state Cruising
    en:
    LMotorVelocity = LDemandVelocity;
    RMotorVelocity = RDemandVelocity;
  (default) -> Idle
  Idle -> Accelerating : [LDemandVelocity ~= 0 && RDemandVelocity ~= 0]{StepTime = CurrentTime}
  Decelerating -> Idle [order 1] : [LMotorVelocity == 0 &&...
      |  RMotorVelocity == 0]
  Accelerating -> Cruising : [LMotorVelocity == LDemandVelocity &&...
      |  RMotorVelocity == RDemandVelocity]
  Cruising -> Accelerating [order 2] : [LDemandVelocity > LMotorVelocity | ...
      | RDemandVelocity > RMotorVelocity]
      | {StepTime = CurrentTime}
  Decelerating -> Cruising [order 2] : [LMotorVelocity == LDemandVelocity &&...
      |  RMotorVelocity == RDemandVelocity]
  Cruising -> Decelerating [commented out] : [DistanceToTarget >- 10 &&...
      | DistanceToTarget < 10]
      | {StepTime = CurrentTime; LDemandVelocity = 0; RDemandVelocity = 0;}
  Cruising -> Decelerating [order 1] : [LDemandVelocity < LMotorVelocity | ...
      | RDemandVelocity < RMotorVelocity]
      | {StepTime = CurrentTime}
  data: CurrentTime function_input; StepTime function_input; TargetVelocity function_input; RampedVelocity function_output; CurrentVelocity function_input; RampRate function_input; LDemandVelocity input single; RDemandVelocity input single; LMotorVelocity output single; RMotorVelocity output single; RampRateA input single; RampRateD input single; CurrentTime input; StepTime local single
  function RampedVelocity = stepToRamp(CurrentTime, StepTime, TargetVelocity, CurrentVelocity, RampRate):
    | function RampedVelocity = stepToRamp(CurrentTime, StepTime, TargetVelocity, CurrentVelocity, RampRate)
    |     % Convert everything to single precision for consistency
    |     CurrentVelocity = single(CurrentVelocity);
    |     TargetVelocity = single(TargetVelocity);
    |     RampRate = single(RampRate);
    |     CurrentTime = single(CurrentTime);
    |     StepTime = single(StepTime);
    |     
    |     % Calculate the remaining velocity to reach the target
    |     VelocityDiff = abs(TargetVelocity - CurrentVelocity);
    |     
    |      % Choose a threshold below which the ramp will smooth (e.g., when within 10% of target)
    |     if TargetVelocity == 0
    |         SmoothingThreshold = single(5);  % Use current velocity for smoothing when target is zero
    |     else
    |         SmoothingThreshold = single(0.1 * abs(TargetVelocity));
    |     end
    | 
    |     if CurrentTime >= StepTime
    |         % Ramping up or down:
    |         if VelocityDiff > SmoothingThreshold
    |             % Standard ramping when far from target
    |             if TargetVelocity > CurrentVelocity
    |                 % Ramping up
    |                 RampedVelocity = single(CurrentVelocity + RampRate * (CurrentTime - StepTime));
    |             else
    |                 % Ramping down
    |                 RampedVelocity = single(CurrentVelocity - RampRate * (CurrentTime - StepTime));
    |             end
    |         else
    |             % Smoothing the ramp as it gets closer to the target velocity
    |             SmoothingFactor = VelocityDiff / SmoothingThreshold;  % Ratio to scale down ramp rate
    |             if TargetVelocity > CurrentVelocity
    |                 % Smoothing ramp up
    |                 RampedVelocity = single(CurrentVelocity + RampRate * SmoothingFactor * (CurrentTime - StepTime));
    |             else
    |                 % Smoothing ramp down
    |                 RampedVelocity = single(CurrentVelocity - RampRate * SmoothingFactor * (CurrentTime - StepTime));
    |             end
    |         end
    | 
    |         % Ensure the velocity doesn't exceed the target velocity in either direction
    |         if TargetVelocity > CurrentVelocity && RampedVelocity > TargetVelocity
    |             RampedVelocity = TargetVelocity;
    |         elseif TargetVelocity < CurrentVelocity && RampedVelocity < TargetVelocity
    |             RampedVelocity = TargetVelocity;
    |         end
    | 
    |     else
    |         % If the step hasn't been applied yet, keep the current velocity
    |         RampedVelocity = CurrentVelocity;
    |     end
    | end
